simulink model "VSC_Simulink"  (R2019b)
settings: Solver=FixedStepDiscrete  StartTime=0.0  StopTime=Inf  FixedStep=T_pwm  MaxStep=1e-4  EnableMultiTasking=on
model workspace (MAT data in the model file):
  Control_P = 0
  Control_PI = 0
  I_integral = 0
  Id_pulse = 0
  Id_ref_const = 0
  Id_simulink = 0
  Id_sin = 0
  Iq_pulse = 0
  Iq_ref_const = 0
  Iq_simulink = 0
  Iq_sin = 0
  K_integral = 0
  K_proporcional = 0
  SELDACB = 0
  SELPWM4A = 0
  SELPWM4B = 0
  SELPWM5A = 0
  SELPWM5B = 0
  SELPWM6A = 0
  SELPWM6B = 0
  a_d = 0
  a_q = 0
  b_integral = 0
  b_proporcional = 0
  open = 0
  open_Id = 0
  open_Iq = 0
  open_control = 0
values from neighbouring files (symbols this model uses):
  Dec = 1    [Sotfware_Matlab.m]
  Frecuencia_Red = 50    [Sotfware_Matlab.m]
  Ib = 2.5    [Sotfware_Matlab.m]
  Ireg_PI = tan((90 + Fc_pi)*pi/180)/wo_pi    [Sotfware_Matlab.m]
  Kreg_P = 1/AP    [Sotfware_Matlab.m]
  Kreg_PI = Ac_pi*Ireg_PI*wo_pi / sqrt(1 + (Ireg_PI*wo_pi)^2)    [Sotfware_Matlab.m]
  Lpu = X_ind/ Lb    [Sotfware_Matlab.m]
  T_pwm = 1/Freq_Conmutacion    (= 0.0001)    [Sotfware_Matlab.m]
  TimerPeriod = Freq_Clock/(Freq_Conmutacion*4)    (= 5000)    [Sotfware_Matlab.m]
  Ub = 0.61*Vdc / sqrt(3)    [Sotfware_Matlab.m]
  w1pu = 1    [Sotfware_Matlab.m]
undefined symbols (not defined in the file or in its folder): Down, GPTRIP1SEL, GPTRIP2SEL, TZ1, TZ2, Up
libraries: c2802xlib x12, c2837xDlib x10, eeTransforms x2, simulink x2
(part 2 of 2)

== system VSC_Simulink/Hardware VSC/Subsystem4 ==
  ADC1 : c2802xlib/ADC  blkParamProc=C2000_Type4  ADCModule=B  samplingMode=Single sample mode  ADCResolution=12-bit (Single-ended input)  useSOC1=SOC5  useSOC2=SOC0_SOC1  SOCAcquisitionWindow=15  SOCTriggerSource=ePWM5_ADCSOCB  SOCInterruptTrigger=No ADCINT  Ts=-1  dType=uint16  postInterrupt=on  interruptSel=ADCINT2  ADCINTContinuous=on  endma=off  chdma=1  conv1=ADCINA0  conv2=ADCINA0 and ADCINB0  conv1_Type4=ADCIN5  conv2_Type4=ADCIN0 and ADCIN1
      settings: SourceProductName=Embedded Coder Support Package for Texas Instruments C2000 Processors
  ADC2 : c2802xlib/ADC  blkParamProc=C2000_Type4  ADCModule=A  samplingMode=Single sample mode  ADCResolution=12-bit (Single-ended input)  useSOC1=SOC5  useSOC2=SOC0_SOC1  SOCAcquisitionWindow=15  SOCTriggerSource=ePWM6_ADCSOCB  SOCInterruptTrigger=No ADCINT  Ts=-1  dType=uint16  postInterrupt=on  interruptSel=ADCINT2  ADCINTContinuous=on  endma=off  chdma=1  conv1=ADCINA0  conv2=ADCINA0 and ADCINB0  conv1_Type4=ADCIN5  conv2_Type4=ADCIN0 and ADCIN1
      settings: SourceProductName=Embedded Coder Support Package for Texas Instruments C2000 Processors
  ADC3 : c2802xlib/ADC  blkParamProc=C2000_Type4  ADCModule=C  samplingMode=Single sample mode  ADCResolution=12-bit (Single-ended input)  useSOC1=SOC4  useSOC2=SOC0_SOC1  SOCAcquisitionWindow=15  SOCTriggerSource=ePWM4_ADCSOCB  SOCInterruptTrigger=No ADCINT  Ts=-1  dType=uint16  postInterrupt=on  interruptSel=ADCINT2  ADCINTContinuous=on  endma=off  chdma=1  conv1=ADCINA0  conv2=ADCINA0 and ADCINB0  conv1_Type4=ADCIN5  conv2_Type4=ADCIN0 and ADCIN1
      settings: SourceProductName=Embedded Coder Support Package for Texas Instruments C2000 Processors
  Out1 : Outport  VectorParamsAs1DForOutWhenUnconnected=off
  Out2 : Outport  Port=2  VectorParamsAs1DForOutWhenUnconnected=off
  Out3 : Outport  Port=3  VectorParamsAs1DForOutWhenUnconnected=off
  wires:
  ADC1/1 -> Out2/1
  ADC2/1 -> Out3/1
  ADC3/1 -> Out1/1

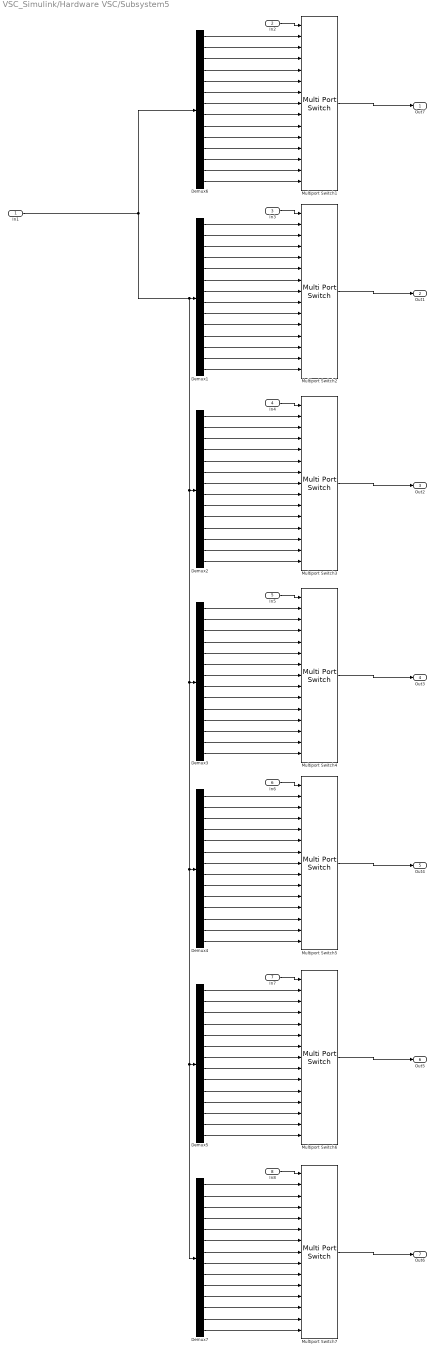
== system VSC_Simulink/Hardware VSC/Subsystem5 ==
  In1 : Inport
  In2 : Inport  Port=2
  In3 : Inport  Port=3
  In4 : Inport  Port=4
  In5 : Inport  Port=5
  In6 : Inport  Port=6
  In7 : Inport  Port=7
  In8 : Inport  Port=8
  Demux{1..7} (7 alike) : Demux  Outputs=14
  Multiport Switch{1..7} (7 alike) : MultiPortSwitch  Inputs=13  DataPortForDefault=Additional data port
  Out7 : Outport  VectorParamsAs1DForOutWhenUnconnected=off
  Out1 : Outport  Port=2  VectorParamsAs1DForOutWhenUnconnected=off
  Out2 : Outport  Port=3  VectorParamsAs1DForOutWhenUnconnected=off
  Out3 : Outport  Port=4  VectorParamsAs1DForOutWhenUnconnected=off
  Out4 : Outport  Port=5  VectorParamsAs1DForOutWhenUnconnected=off
  Out5 : Outport  Port=6  VectorParamsAs1DForOutWhenUnconnected=off
  Out6 : Outport  Port=7  VectorParamsAs1DForOutWhenUnconnected=off
  wires:
  In1/1 -> Demux7/1, Demux5/1, Demux4/1, Demux3/1, Demux2/1, Demux1/1, Demux6/1
  In2/1 -> Multiport Switch1/1
  Demux6/9 -> Multiport Switch1/10
  Demux6/8 -> Multiport Switch1/9
  Demux6/7 -> Multiport Switch1/8
  Demux6/6 -> Multiport Switch1/7
  Demux6/4 -> Multiport Switch1/5
  Demux6/5 -> Multiport Switch1/6
  Demux6/3 -> Multiport Switch1/4
  Demux6/2 -> Multiport Switch1/3
  Demux6/1 -> Multiport Switch1/2
  Multiport Switch1/1 -> Out7/1
  Demux6/10 -> Multiport Switch1/11
  Demux6/11 -> Multiport Switch1/12
  Demux6/13 -> Multiport Switch1/14
  Demux6/14 -> Multiport Switch1/15
  Demux6/12 -> Multiport Switch1/13
  Demux1/12 -> Multiport Switch2/13
  Demux1/14 -> Multiport Switch2/15
  Demux1/13 -> Multiport Switch2/14
  Demux1/11 -> Multiport Switch2/12
  Demux1/10 -> Multiport Switch2/11
  Multiport Switch2/1 -> Out1/1
  Demux1/1 -> Multiport Switch2/2
  Demux1/2 -> Multiport Switch2/3
  Demux1/3 -> Multiport Switch2/4
  Demux1/5 -> Multiport Switch2/6
  Demux1/4 -> Multiport Switch2/5
  Demux1/6 -> Multiport Switch2/7
  Demux1/7 -> Multiport Switch2/8
  Demux1/8 -> Multiport Switch2/9
  Demux1/9 -> Multiport Switch2/10
  In3/1 -> Multiport Switch2/1
  In4/1 -> Multiport Switch3/1
  Demux2/9 -> Multiport Switch3/10
  Demux2/8 -> Multiport Switch3/9
  Demux2/7 -> Multiport Switch3/8
  Demux2/6 -> Multiport Switch3/7
  Demux2/4 -> Multiport Switch3/5
  Demux2/5 -> Multiport Switch3/6
  Demux2/3 -> Multiport Switch3/4
  Demux2/2 -> Multiport Switch3/3
  Demux2/1 -> Multiport Switch3/2
  Multiport Switch3/1 -> Out2/1
  Demux2/10 -> Multiport Switch3/11
  Demux2/11 -> Multiport Switch3/12
  Demux2/13 -> Multiport Switch3/14
  Demux2/14 -> Multiport Switch3/15
  Demux2/12 -> Multiport Switch3/13
  Demux3/12 -> Multiport Switch4/13
  Demux3/14 -> Multiport Switch4/15
  Demux3/13 -> Multiport Switch4/14
  Demux3/11 -> Multiport Switch4/12
  Demux3/10 -> Multiport Switch4/11
  Multiport Switch4/1 -> Out3/1
  Demux3/1 -> Multiport Switch4/2
  Demux3/2 -> Multiport Switch4/3
  Demux3/3 -> Multiport Switch4/4
  Demux3/5 -> Multiport Switch4/6
  Demux3/4 -> Multiport Switch4/5
  Demux3/6 -> Multiport Switch4/7
  Demux3/7 -> Multiport Switch4/8
  Demux3/8 -> Multiport Switch4/9
  Demux3/9 -> Multiport Switch4/10
  In5/1 -> Multiport Switch4/1
  In6/1 -> Multiport Switch5/1
  Demux4/9 -> Multiport Switch5/10
  Demux4/8 -> Multiport Switch5/9
  Demux4/7 -> Multiport Switch5/8
  Demux4/6 -> Multiport Switch5/7
  Demux4/4 -> Multiport Switch5/5
  Demux4/5 -> Multiport Switch5/6
  Demux4/3 -> Multiport Switch5/4
  Demux4/2 -> Multiport Switch5/3
  Demux4/1 -> Multiport Switch5/2
  Multiport Switch5/1 -> Out4/1
  Demux4/10 -> Multiport Switch5/11
  Demux4/11 -> Multiport Switch5/12
  Demux4/13 -> Multiport Switch5/14
  Demux4/14 -> Multiport Switch5/15
  Demux4/12 -> Multiport Switch5/13
  Demux5/12 -> Multiport Switch6/13
  Demux5/14 -> Multiport Switch6/15
  Demux5/13 -> Multiport Switch6/14
  Demux5/11 -> Multiport Switch6/12
  Demux5/10 -> Multiport Switch6/11
  Multiport Switch6/1 -> Out5/1
  Demux5/1 -> Multiport Switch6/2
  Demux5/2 -> Multiport Switch6/3
  Demux5/3 -> Multiport Switch6/4
  Demux5/5 -> Multiport Switch6/6
  Demux5/4 -> Multiport Switch6/5
  Demux5/6 -> Multiport Switch6/7
  Demux5/7 -> Multiport Switch6/8
  Demux5/8 -> Multiport Switch6/9
  Demux5/9 -> Multiport Switch6/10
  In7/1 -> Multiport Switch6/1
  In8/1 -> Multiport Switch7/1
  Demux7/9 -> Multiport Switch7/10
  Demux7/8 -> Multiport Switch7/9
  Demux7/7 -> Multiport Switch7/8
  Demux7/6 -> Multiport Switch7/7
  Demux7/4 -> Multiport Switch7/5
  Demux7/5 -> Multiport Switch7/6
  Demux7/3 -> Multiport Switch7/4
  Demux7/2 -> Multiport Switch7/3
  Demux7/1 -> Multiport Switch7/2
  Multiport Switch7/1 -> Out6/1
  Demux7/10 -> Multiport Switch7/11
  Demux7/11 -> Multiport Switch7/12
  Demux7/13 -> Multiport Switch7/14
  Demux7/14 -> Multiport Switch7/15
  Demux7/12 -> Multiport Switch7/13

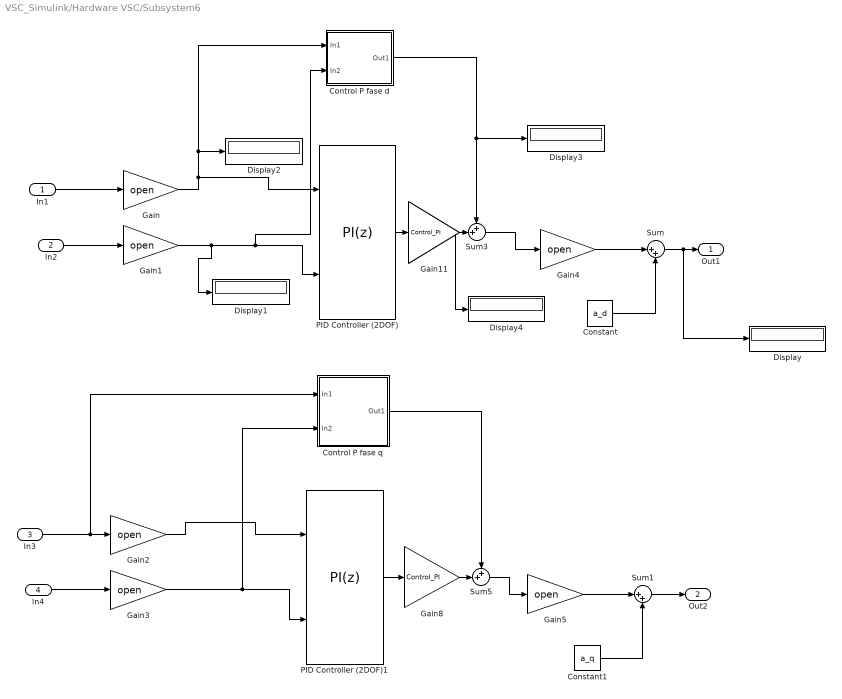
== system VSC_Simulink/Hardware VSC/Subsystem6 ==
  In1 : Inport
  In2 : Inport  Port=2
  In3 : Inport  Port=3
  In4 : Inport  Port=4
  Constant : Constant  Value=a_d
  Constant1 : Constant  Value=a_q
  Control P fase d : Subsystem
  Control P fase q : Subsystem
  Display{,1..4} (5 alike) : Display
  Gain{,1..5} (6 alike) : Gain  Gain=open
  Gain11 : Gain  Gain=Control_PI
  Gain8 : Gain  Gain=Control_PI
  PID Controller (2DOF) : simulink/Continuous/PID Controller (2DOF)  Controller=PI  Form=Ideal  TimeDomain=Discrete-time  SampleTime=-1  IntegratorMethod=Forward Euler  FilterMethod=Forward Euler  ControllerParametersSource=internal  P=K_integral  I=K_integral/I_integral  D=0  UseFilter=on  N=100  b=b_integral  c=1  TunerSelectOption=Frequency Response Based  InitialConditionSource=internal  InitialConditionForIntegrator=0  InitialConditionForFilter=0  DifferentiatorICPrevScaledInput=0  ExternalReset=none  TrackingMode=off  Kt=1  LimitOutput=off  UpperSaturationLimit=1.5  LowerSaturationLimit=-3  LinearizeAsGain=on  AntiWindupMode=none  Kb=1  POutMin=[]  POutMax=[]  IOutMin=[]  IOutMax=[]  DOutMin=[]  DOutMax=[]  NOutMin=[]  NOutMax=[]  bOutMin=[]  bOutMax=[]  cOutMin=[]  cOutMax=[]  SumOutMin=[]  SumOutMax=[]  SaturationOutMin=[]  SaturationOutMax=[]  PParamMin=[]  PParamMax=[]  IParamMin=[]  IParamMax=[]  DParamMin=[]  DParamMax=[]  NParamMin=[]  NParamMax=[]  bParamMin=[]  bParamMax=[]  cParamMin=[]  cParamMax=[]  KbParamMin=[]  KbParamMax=[]  KtParamMin=[]  KtParamMax=[]  KbOutMin=[]  KbOutMax=[]  KtOutMin=[]  KtOutMax=[]  IntegratorOutMin=[]  IntegratorOutMax=[]  FilterOutMin=[]  FilterOutMax=[]  SumI1OutMin=[]  SumI1OutMax=[]  SumI2OutMin=[]  SumI2OutMax=[]  SumI3OutMin=[]  SumI3OutMax=[]  SumI4OutMin=[]  SumI4OutMax=[]  SumDOutMin=[]  SumDOutMax=[]  Sum1OutMin=[]  Sum1OutMax=[]  Sum2OutMin=[]  Sum2OutMax=[]  Sum3OutMin=[]  Sum3OutMax=[]  DifferentiatorOutMin=[]  DifferentiatorOutMax=[]  FilterDiffOutCoefMin=[]  FilterDiffOutCoefMax=[]  ReciprocalOutMin=[]  ReciprocalOutMax=[]  SumDenOutMin=[]  SumDenOutMax=[]  SumNumOutMin=[]  SumNumOutMax=[]  DivideOutMin=[]  DivideOutMax=[]  IntegratorContinuousStateAttributes=''  IntegratorStateMustResolveToSignalObject=off  IntegratorRTWStateStorageClass=Auto  FilterContinuousStateAttributes=''  FilterStateMustResolveToSignalObject=off  FilterRTWStateStorageClass=Auto  ParallelPVariant=Passthrough  IdealPVariant=InternalParameters  IVariant=InternalParameters  DVariant=Disabled  bVariant=InternalParameters  cVariant=Disabled  IntegratorVariant=Discrete  SatVariant=Disabled  AWVariant=Passthrough  PCopyVariant=Disabled  TRVariant=Disabled  FdbkBlocksVariant=Forward  IdealPFdbkVariant=Disabled  SatFdbkVariant=Disabled  DerivativeFilterVariant=Disabled  NVariant=Disabled  NCopyVariant=Disabled_SignalSpec  FilterICVariant=Disabled  IntegratorICVariant=InternalICs  ExternalResetVariant=Disabled  TRSumVariant=Passthrough  SumFdbkVariant=Disabled  SumVariant=Sum_PI
  PID Controller (2DOF)1 : simulink/Continuous/PID Controller (2DOF)  Controller=PI  Form=Ideal  TimeDomain=Discrete-time  SampleTime=-1  IntegratorMethod=Forward Euler  FilterMethod=Forward Euler  ControllerParametersSource=internal  P=K_integral  I=K_integral/I_integral  D=0  UseFilter=on  N=100  b=b_integral  c=1  TunerSelectOption=Frequency Response Based  InitialConditionSource=internal  InitialConditionForIntegrator=0  InitialConditionForFilter=0  DifferentiatorICPrevScaledInput=0  ExternalReset=none  TrackingMode=off  Kt=1  LimitOutput=off  UpperSaturationLimit=1.5  LowerSaturationLimit=-3  LinearizeAsGain=on  AntiWindupMode=none  Kb=1  POutMin=[]  POutMax=[]  IOutMin=[]  IOutMax=[]  DOutMin=[]  DOutMax=[]  NOutMin=[]  NOutMax=[]  bOutMin=[]  bOutMax=[]  cOutMin=[]  cOutMax=[]  SumOutMin=[]  SumOutMax=[]  SaturationOutMin=[]  SaturationOutMax=[]  PParamMin=[]  PParamMax=[]  IParamMin=[]  IParamMax=[]  DParamMin=[]  DParamMax=[]  NParamMin=[]  NParamMax=[]  bParamMin=[]  bParamMax=[]  cParamMin=[]  cParamMax=[]  KbParamMin=[]  KbParamMax=[]  KtParamMin=[]  KtParamMax=[]  KbOutMin=[]  KbOutMax=[]  KtOutMin=[]  KtOutMax=[]  IntegratorOutMin=[]  IntegratorOutMax=[]  FilterOutMin=[]  FilterOutMax=[]  SumI1OutMin=[]  SumI1OutMax=[]  SumI2OutMin=[]  SumI2OutMax=[]  SumI3OutMin=[]  SumI3OutMax=[]  SumI4OutMin=[]  SumI4OutMax=[]  SumDOutMin=[]  SumDOutMax=[]  Sum1OutMin=[]  Sum1OutMax=[]  Sum2OutMin=[]  Sum2OutMax=[]  Sum3OutMin=[]  Sum3OutMax=[]  DifferentiatorOutMin=[]  DifferentiatorOutMax=[]  FilterDiffOutCoefMin=[]  FilterDiffOutCoefMax=[]  ReciprocalOutMin=[]  ReciprocalOutMax=[]  SumDenOutMin=[]  SumDenOutMax=[]  SumNumOutMin=[]  SumNumOutMax=[]  DivideOutMin=[]  DivideOutMax=[]  IntegratorContinuousStateAttributes=''  IntegratorStateMustResolveToSignalObject=off  IntegratorRTWStateStorageClass=Auto  FilterContinuousStateAttributes=''  FilterStateMustResolveToSignalObject=off  FilterRTWStateStorageClass=Auto  ParallelPVariant=Passthrough  IdealPVariant=InternalParameters  IVariant=InternalParameters  DVariant=Disabled  bVariant=InternalParameters  cVariant=Disabled  IntegratorVariant=Discrete  SatVariant=Disabled  AWVariant=Passthrough  PCopyVariant=Disabled  TRVariant=Disabled  FdbkBlocksVariant=Forward  IdealPFdbkVariant=Disabled  SatFdbkVariant=Disabled  DerivativeFilterVariant=Disabled  NVariant=Disabled  NCopyVariant=Disabled_SignalSpec  FilterICVariant=Disabled  IntegratorICVariant=InternalICs  ExternalResetVariant=Disabled  TRSumVariant=Passthrough  SumFdbkVariant=Disabled  SumVariant=Sum_PI
  Sum : Sum  Inputs=|++
  Sum1 : Sum  Inputs=|++
  Sum3 : Sum  Inputs=++|
  Sum5 : Sum  Inputs=++|
  Out1 : Outport  VectorParamsAs1DForOutWhenUnconnected=off
  Out2 : Outport  Port=2  VectorParamsAs1DForOutWhenUnconnected=off
  wires:
  Gain4/1 -> Sum/1
  In3/1 -> Control P fase q/1(In1), Gain2/1
  PID Controller (2DOF)/1 -> Gain11/1
  Constant/1 -> Sum/2
  Gain3/1 -> Control P fase q/2(In2), PID Controller (2DOF)1/2
  In2/1 -> Gain1/1
  Gain/1 -> Control P fase d/1(In1), Display2/1, PID Controller (2DOF)/1
  Gain1/1 -> Display1/1, Control P fase d/2(In2), PID Controller (2DOF)/2
  PID Controller (2DOF)1/1 -> Gain8/1
  Sum/1 -> Display/1, Out1/1
  In4/1 -> Gain3/1
  Gain8/1 -> Sum5/2
  Gain2/1 -> PID Controller (2DOF)1/1
  In1/1 -> Gain/1
  Sum1/1 -> Out2/1
  Gain11/1 -> Display4/1, Sum3/2
  Sum5/1 -> Gain5/1
  Constant1/1 -> Sum1/2
  Gain5/1 -> Sum1/1
  Sum3/1 -> Gain4/1
  Control P fase q/1(Out1) -> Sum5/1
  Control P fase d/1(Out1) -> Display3/1, Sum3/1

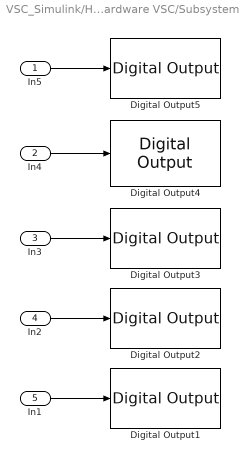
== system VSC_Simulink/Hardware VSC/Subsystem7 ==
  In5 : Inport
  In4 : Inport  Port=2
  In3 : Inport  Port=3
  In2 : Inport  Port=4
  In1 : Inport  Port=5
  Digital Output1 : c2837xDlib/Digital Output  GPIO_Number=GPIO56~GPIO63  GPIO_Bit0=off  GPIO_BIT0_Toggle=off  GPIO_Bit1=off  GPIO_BIT1_Toggle=off  GPIO_Bit2=on  GPIO_BIT2_Toggle=off  GPIO_Bit3=off  GPIO_BIT3_Toggle=off  GPIO_Bit4=off  GPIO_BIT4_Toggle=off  GPIO_Bit5=off  GPIO_BIT5_Toggle=off  GPIO_Bit6=off  GPIO_BIT6_Toggle=off  GPIO_Bit7=off  GPIO_BIT7_Toggle=off
      settings: SourceProductName=Embedded Coder Support Package for Texas Instruments C2000 Processors  SourceProductBaseCode=TIC2000
  Digital Output2 : c2837xDlib/Digital Output  GPIO_Number=GPIO56~GPIO63  GPIO_Bit0=off  GPIO_BIT0_Toggle=off  GPIO_Bit1=off  GPIO_BIT1_Toggle=off  GPIO_Bit2=off  GPIO_BIT2_Toggle=off  GPIO_Bit3=on  GPIO_BIT3_Toggle=off  GPIO_Bit4=off  GPIO_BIT4_Toggle=off  GPIO_Bit5=off  GPIO_BIT5_Toggle=off  GPIO_Bit6=off  GPIO_BIT6_Toggle=off  GPIO_Bit7=off  GPIO_BIT7_Toggle=off
      settings: SourceProductName=Embedded Coder Support Package for Texas Instruments C2000 Processors  SourceProductBaseCode=TIC2000
  Digital Output3 : c2837xDlib/Digital Output  GPIO_Number=GPIO120~GPIO127  GPIO_Bit0=off  GPIO_BIT0_Toggle=off  GPIO_Bit1=off  GPIO_BIT1_Toggle=off  GPIO_Bit2=off  GPIO_BIT2_Toggle=off  GPIO_Bit3=off  GPIO_BIT3_Toggle=off  GPIO_Bit4=on  GPIO_BIT4_Toggle=off  GPIO_Bit5=off  GPIO_BIT5_Toggle=off  GPIO_Bit6=off  GPIO_BIT6_Toggle=off  GPIO_Bit7=off  GPIO_BIT7_Toggle=off
      settings: SourceProductName=Embedded Coder Support Package for Texas Instruments C2000 Processors  SourceProductBaseCode=TIC2000
  Digital Output4 : c2837xDlib/Digital Output  GPIO_Number=GPIO120~GPIO127  GPIO_Bit0=off  GPIO_BIT0_Toggle=off  GPIO_Bit1=off  GPIO_BIT1_Toggle=off  GPIO_Bit2=off  GPIO_BIT2_Toggle=off  GPIO_Bit3=off  GPIO_BIT3_Toggle=off  GPIO_Bit4=off  GPIO_BIT4_Toggle=off  GPIO_Bit5=on  GPIO_BIT5_Toggle=off  GPIO_Bit6=off  GPIO_BIT6_Toggle=off  GPIO_Bit7=off  GPIO_BIT7_Toggle=off
      settings: SourceProductName=Embedded Coder Support Package for Texas Instruments C2000 Processors  SourceProductBaseCode=TIC2000
  Digital Output5 : c2837xDlib/Digital Output  GPIO_Number=GPIO24~GPIO31  GPIO_Bit0=off  GPIO_BIT0_Toggle=off  GPIO_Bit1=off  GPIO_BIT1_Toggle=off  GPIO_Bit2=off  GPIO_BIT2_Toggle=off  GPIO_Bit3=off  GPIO_BIT3_Toggle=off  GPIO_Bit4=off  GPIO_BIT4_Toggle=off  GPIO_Bit5=on  GPIO_BIT5_Toggle=off  GPIO_Bit6=off  GPIO_BIT6_Toggle=off  GPIO_Bit7=off  GPIO_BIT7_Toggle=off
      settings: SourceProductName=Embedded Coder Support Package for Texas Instruments C2000 Processors  SourceProductBaseCode=TIC2000
  wires:
  In1/1 -> Digital Output1/1
  In2/1 -> Digital Output2/1
  In3/1 -> Digital Output3/1
  In4/1 -> Digital Output4/1
  In5/1 -> Digital Output5/1

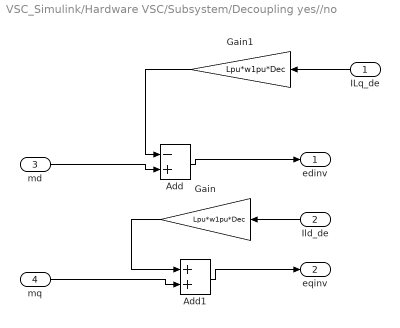
== system VSC_Simulink/Hardware VSC/Subsystem/Decoupling yes//no ==
  ILq_de : Inport
  Ild_de : Inport  Port=2
  md : Inport  Port=3
  mq : Inport  Port=4
  Add : Sum  Inputs=-+
  Add1 : Sum
  Gain : Gain  Gain=Lpu*w1pu*Dec
  Gain1 : Gain  Gain=Lpu*w1pu*Dec
  edinv : Outport  VectorParamsAs1DForOutWhenUnconnected=off
  eqinv : Outport  Port=2  VectorParamsAs1DForOutWhenUnconnected=off
  wires:
  Add1/1 -> eqinv/1
  ILq_de/1 -> Gain1/1
  mq/1 -> Add1/2
  Gain1/1 -> Add/1
  Ild_de/1 -> Gain/1
  Gain/1 -> Add1/1
  Add/1 -> edinv/1
  md/1 -> Add/2

== system VSC_Simulink/Hardware VSC/Subsystem3/DAC1 ==
  In1 : Inport
  Constant8 : Constant  Value=2048  SampleTime=-1
  DAC2 : c2837xDlib/DAC  channel=A  saturate=off
      settings: SourceProductName=Embedded Coder Support Package for Texas Instruments C2000 Processors  SourceProductBaseCode=TIC2000
  Gain : Gain  Gain=2048
  Gain1 : Gain  Gain=0.5
  Sum1 : Sum  Inputs=|++
  wires:
  Constant8/1 -> Sum1/2
  Gain/1 -> Sum1/1
  Sum1/1 -> DAC2/1
  In1/1 -> Gain1/1
  Gain1/1 -> Gain/1

== system VSC_Simulink/Hardware VSC/Subsystem6/Control P fase d ==
  In1 : Inport
  In2 : Inport  Port=2
  Gain10 : Gain  Gain=Control_P
  Gain6 : Gain  Gain=K_proporcional
  Sum2 : Sum  Inputs=|+-
  Out1 : Outport  VectorParamsAs1DForOutWhenUnconnected=off
  wires:
  In1/1 -> Sum2/1
  Gain10/1 -> Out1/1
  In2/1 -> Gain6/1
  Sum2/1 -> Gain10/1
  Gain6/1 -> Sum2/2

== system VSC_Simulink/Hardware VSC/Subsystem6/Control P fase q ==
  In1 : Inport
  In2 : Inport  Port=2
  Gain7 : Gain  Gain=K_proporcional
  Gain9 : Gain  Gain=Control_P
  Sum4 : Sum  Inputs=|+-
  Out1 : Outport  VectorParamsAs1DForOutWhenUnconnected=off
  wires:
  Gain9/1 -> Out1/1
  In2/1 -> Gain7/1
  Sum4/1 -> Gain9/1
  In1/1 -> Sum4/1
  Gain7/1 -> Sum4/2
